simulink model "left_leg"  (R2017b)
settings: Solver=FixedStepAuto  StartTime=0.0  StopTime=inf  RelTol=1e-3  EnableMultiTasking=on
libraries: ComponentLibrary x6
settings Model: xpc_rtwmakecfg_data=_xpcethercatlib_  SimulationMode=external  Creator=hanli  LastModifiedBy=hanli
settings SolverCC: ConcurrentTasks=on  AutoInsertRateTranBlk=on
settings DataIOCC: SaveFormat=StructureWithTime
settings OptimizationCC: BlockReduction=off  OptimizeBlockIOStorage=off  BufferReuse=off  GlobalBufferReuse=off  ExpressionFolding=off  LocalBlockOutputs=off
settings HardwareCC: ProdBitPerPointer=32  ProdBitPerSizeT=32  ProdBitPerPtrDiffT=32  ProdLargestAtomicFloat=None  ProdWordSize=32  ProdLongLongMode=on  ProdHWDeviceType=Generic->32-bit x86 compatible
settings RTWCC: SystemTargetFile=slrt.tlc  TemplateMakefile=slrt_default_tmf  Description=Simulink Real-Time  CodeExecutionProfiling=on  RTWCompilerOptimization=on
settings SimulinkRealTimeCC: SupportVariableSizeSignals=on  RL32LogTETModifier=off  xPCConcurrentTasks=on

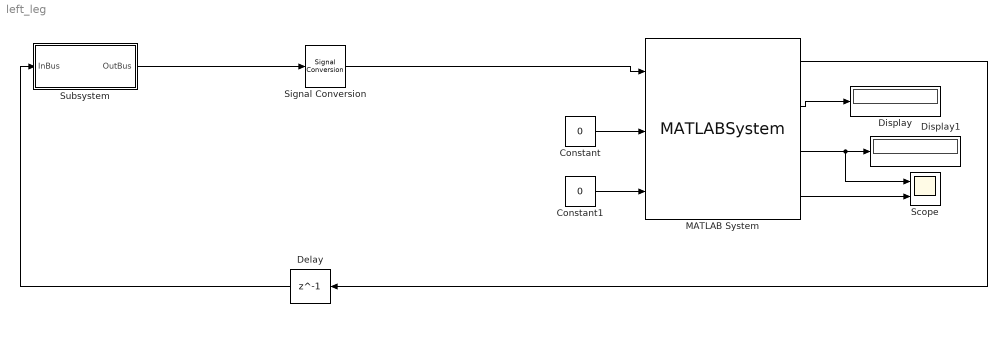
== system left_leg ==
  Constant : Constant  Value=0  OutDataTypeStr=double
  Constant1 : Constant  Value=0  OutDataTypeStr=double
  Delay : Delay  DelayLength=1  InitialCondition=0
  Display : Display
      settings: Format=short_e
  Display1 : Display
  MATLAB System : MATLABSystem  System=Controller_s  SimulateUsing=Code generation
      mask Type: Controller_s
      mask Display:
      | disp('Controller_s');
      | port_label('input',1,'cassieOutputs');
      | port_label('input',2,'p_val');
      | port_label('input',3,'d_val');
      | port_label('output',1,'userInputs');
      | port_label('output',2,'error_rms');
      | port_label('output',3,'real_val');
      | port_label('output',4,'actual_val');
  Scope : Scope  NumInputPorts=2
  Signal Conversion : SignalConversion  ConversionOutput=Nonvirtual bus  OutDataTypeStr=Bus: CassieOutBus  OverrideOpt=off
  Subsystem : Subsystem
  wires:
  Delay/1 -> Subsystem/1(InBus)
  Signal Conversion/1 -> MATLAB System/1
  Subsystem/1(OutBus) -> Signal Conversion/1
  Constant1/1 -> MATLAB System/3
  Constant/1 -> MATLAB System/2
  MATLAB System/2 -> Display/1
  MATLAB System/1 -> Delay/1
  MATLAB System/3 -> Display1/1, Scope/1
  MATLAB System/4 -> Scope/2

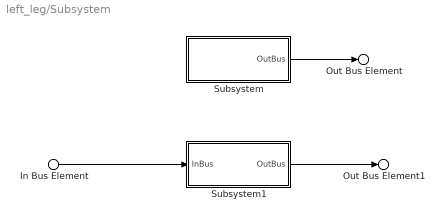
== system left_leg/Subsystem ==
  In Bus Element : Inport  PortName=InBus  Element=leftLeg
  Subsystem : Subsystem
  Subsystem1 : Subsystem
  Out Bus Element : Outport  PortName=OutBus  Element=pelvis
  Out Bus Element1 : Outport  PortName=OutBus  Element=leftLeg
  wires:
  Subsystem/1(OutBus) -> Out Bus Element/1
  In Bus Element/1 -> Subsystem1/1(InBus)
  Subsystem1/1(OutBus) -> Out Bus Element1/1

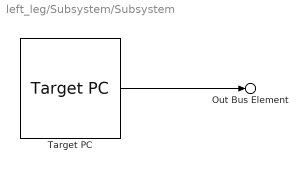
== system left_leg/Subsystem/Subsystem ==
  Target PC : ComponentLibrary/RealTime/Target PC  config_file=C:\Users\hanli\Desktop\robot\Controllers\test_one_leg\xml\l.xml  pci_bus=1  pci_slot=0  pci_function=0
      link override EtherCAT Init: sample_time=0.000500  DCMode=2
  Out Bus Element : Outport  PortName=OutBus  Element=targetPc
  wires:
  Target PC/1 -> Out Bus Element/1

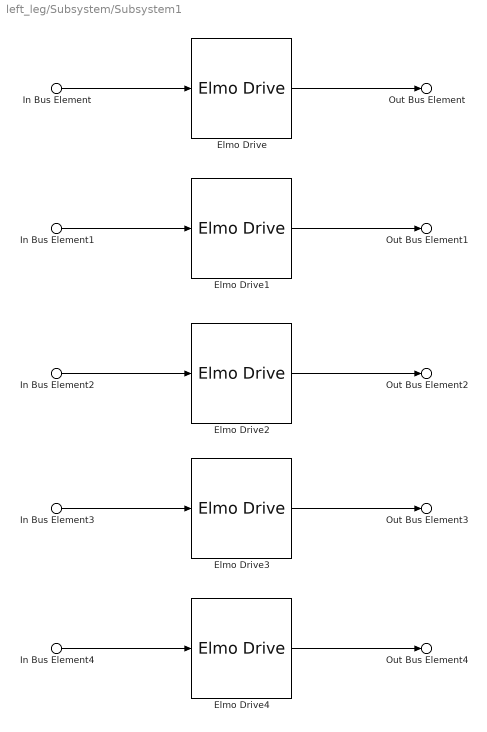
== system left_leg/Subsystem/Subsystem1 ==
  In Bus Element4 : Inport  PortName=InBus  Element=footDrive
  In Bus Element : Inport  PortName=InBus  Element=hipRollDrive
  In Bus Element1 : Inport  PortName=InBus  Element=hipYawDrive
  In Bus Element2 : Inport  PortName=InBus  Element=hipPitchDrive
  In Bus Element3 : Inport  PortName=InBus  Element=kneeDrive
  Elmo Drive : ComponentLibrary/RealTime/Elmo Drive  ethercatName=hipRollDrive  slaveAddress=1001  currentLimit=11.3  gearRatio=1  encoderCounts=2^19  Offset=46574
      link override Control Word PDO Transmit: sig_name=hipRollDrive.Outputs.Control word  sig_offset=2144  sample_time=0.001000
      link override Mode of Operation PDO Transmit: sig_name=hipRollDrive.Outputs.Modes of operation  sig_offset=480  sig_type=int8  type_size=8  sample_time=0.0005
      link override Status Word PDO Receive: sample_time=0.0005
  Elmo Drive1 : ComponentLibrary/RealTime/Elmo Drive  ethercatName=hipYawDrive  slaveAddress=1002  currentLimit=11.3  gearRatio=1  encoderCounts=2^19  Offset=483452
  Elmo Drive2 : ComponentLibrary/RealTime/Elmo Drive  ethercatName=hipPitchDrive  slaveAddress=1003  currentLimit=15.55  gearRatio=1  encoderCounts=2^20  Offset=704266
  Elmo Drive3 : ComponentLibrary/RealTime/Elmo Drive  ethercatName=kneeDrive  slaveAddress=1004  currentLimit=15.55  gearRatio=1  encoderCounts=2^20  Offset=662872
  Elmo Drive4 : ComponentLibrary/RealTime/Elmo Drive  ethercatName=footDrive  slaveAddress=1005  currentLimit=7  gearRatio=1  encoderCounts=2^19  Offset=331361
  Out Bus Element : Outport  PortName=OutBus  Element=hipRollDrive
  Out Bus Element1 : Outport  PortName=OutBus  Element=hipYawDrive
  Out Bus Element2 : Outport  PortName=OutBus  Element=hipPitchDrive
  Out Bus Element3 : Outport  PortName=OutBus  Element=kneeDrive
  Out Bus Element4 : Outport  PortName=OutBus  Element=footDrive
  wires:
  In Bus Element/1 -> Elmo Drive/1
  Elmo Drive/1 -> Out Bus Element/1
  In Bus Element1/1 -> Elmo Drive1/1
  Elmo Drive1/1 -> Out Bus Element1/1
  In Bus Element2/1 -> Elmo Drive2/1
  Elmo Drive2/1 -> Out Bus Element2/1
  In Bus Element3/1 -> Elmo Drive3/1
  Elmo Drive3/1 -> Out Bus Element3/1
  Elmo Drive4/1 -> Out Bus Element4/1
  In Bus Element4/1 -> Elmo Drive4/1
